simulink model "Timer"  (R2022a)
settings: Solver=ode3  StartTime=0.0  StopTime=10.0  FixedStep=0.01  RelTol=1e-3  EnableMultiTasking=on
settings Model: Creator=60251  LastModifiedBy=60251
settings SolverCC: AlgebraicLoopSolver=TrustRegion
settings DebuggingCC: UnconnectedInputMsg=warning  UnconnectedOutputMsg=warning  UnconnectedLineMsg=warning  SFMachineParentedDataDiag=warning
settings RTWCC: DLArmComputeVersion=19.05

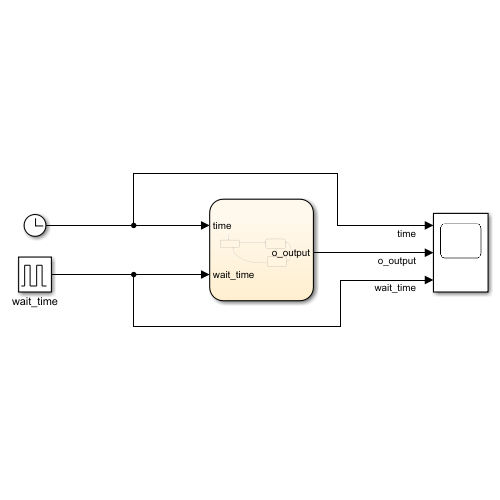
[thumbnail: Simulink's stored preview of the top-level diagram]
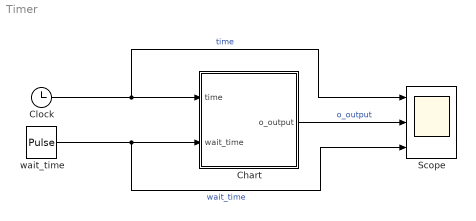
== system Timer ==
  Chart : Stateflow chart  TreatAsAtomicUnit=on
  Clock : Clock
  Scope : Scope  NumInputPorts=3
  wait_time : DiscretePulseGenerator  PulseType=Time based  Period=3  PulseWidth=50
  wires:
  Clock/1 -> Chart/1(time), Scope/1  "time"
  wait_time/1 -> Scope/3, Chart/2(wait_time)  "wait_time"
  Chart/1(o_output) -> Scope/2  "o_output"

== stateflow chart Timer/Chart ==
  state Warten
    en: t = time;
    en: wait = wait_time;
    ex: o_output = 1;
    %exit=Verlassen
  state Null
    en: o_output = 0;
    %entry=Eintritt
  note: ungleichheit
  state Check
    ex: o_output = 0
  (default) -> Null
  Check -> Warten [order 1] : [wait_time ~= 0]
  Null -> Warten : [wait_time ~= 0]
  Check -> Null [order 2] : [wait_time == 0]
  Warten -> Check : [time-(t+wait) >= 0]
  data: time input; wait_time input; o_output output; wait local; t local
